simulink model "thermal_stress_control_gpu"  (R2025b)
settings: Solver=FixedStepDiscrete  StartTime=0.0  StopTime=40.0  FixedStep=0.05  RelTol=1e-3
undefined symbols (not defined in the file or in its folder): DiscIntNeverNeededParam
settings Model: Creator=fbetancourt  LastModifiedBy=fbetancourt

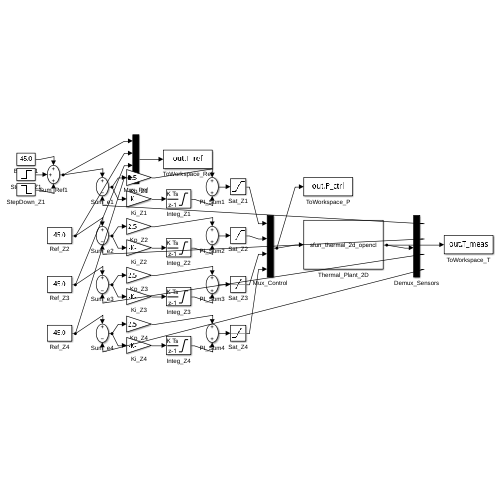
[thumbnail: Simulink's stored preview of the top-level diagram]
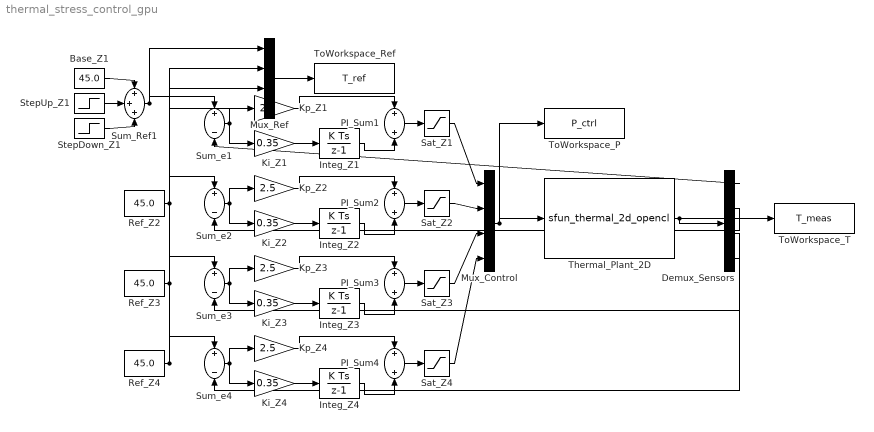
== system thermal_stress_control_gpu ==
  Base_Z1 : Constant  Value=45.0  SampleTime=0.05
  Demux_Sensors : Demux
  Integ_Z{1..4} (4 alike) : DiscreteIntegrator  SampleTime=0.05  LimitOutput=on  UpperSaturationLimit=100.0  LowerSaturationLimit=0.0  ICPrevOutput=DiscIntNeverNeededParam  ICPrevScaledInput=DiscIntNeverNeededParam
  Ki_Z{1..4} (4 alike) : Gain  Gain=0.35
  Kp_Z{1..4} (4 alike) : Gain  Gain=2.5
  Mux_Control : Mux
  Mux_Ref : Mux
  PI_Sum{1..4} (4 alike) : Sum
  Ref_Z2 : Constant  Value=45.0  SampleTime=0.05
  Ref_Z3 : Constant  Value=45.0  SampleTime=0.05
  Ref_Z4 : Constant  Value=45.0  SampleTime=0.05
  Sat_Z{1..4} (4 alike) : Saturate  UpperLimit=100.0  LowerLimit=0.0
  StepDown_Z1 : Step  Time=24.0  Before=0.0  After=-65.0  SampleTime=0.05
  StepUp_Z1 : Step  Time=8.0  Before=0.0  After=65.0  SampleTime=0.05
  Sum_Ref1 : Sum  Inputs=+++
  Sum_e{1..4} (4 alike) : Sum  Inputs=+-
  Thermal_Plant_2D : S-Function  FunctionName=sfun_thermal_2d_opencl  SFunctionDeploymentMode=off  EnableBusSupport=off
  ToWorkspace_P : ToWorkspace  VariableName=P_ctrl  SampleTime=0.05
  ToWorkspace_Ref : ToWorkspace  VariableName=T_ref  SampleTime=0.05
  ToWorkspace_T : ToWorkspace  VariableName=T_meas  SampleTime=0.05
  wires:
  Mux_Control/1 -> Thermal_Plant_2D/1, ToWorkspace_P/1
  Thermal_Plant_2D/1 -> Demux_Sensors/1, ToWorkspace_T/1
  Base_Z1/1 -> Sum_Ref1/1
  StepUp_Z1/1 -> Sum_Ref1/2
  StepDown_Z1/1 -> Sum_Ref1/3
  Sum_Ref1/1 -> Mux_Ref/1, Sum_e1/1
  Demux_Sensors/1 -> Sum_e1/2
  Sum_e1/1 -> Kp_Z1/1, Ki_Z1/1
  Ki_Z1/1 -> Integ_Z1/1
  Kp_Z1/1 -> PI_Sum1/1
  Integ_Z1/1 -> PI_Sum1/2
  PI_Sum1/1 -> Sat_Z1/1
  Sat_Z1/1 -> Mux_Control/1
  Ref_Z2/1 -> Mux_Ref/2, Sum_e2/1
  Demux_Sensors/2 -> Sum_e2/2
  Sum_e2/1 -> Kp_Z2/1, Ki_Z2/1
  Ki_Z2/1 -> Integ_Z2/1
  Kp_Z2/1 -> PI_Sum2/1
  Integ_Z2/1 -> PI_Sum2/2
  PI_Sum2/1 -> Sat_Z2/1
  Sat_Z2/1 -> Mux_Control/2
  Ref_Z3/1 -> Mux_Ref/3, Sum_e3/1
  Demux_Sensors/3 -> Sum_e3/2
  Sum_e3/1 -> Kp_Z3/1, Ki_Z3/1
  Ki_Z3/1 -> Integ_Z3/1
  Kp_Z3/1 -> PI_Sum3/1
  Integ_Z3/1 -> PI_Sum3/2
  PI_Sum3/1 -> Sat_Z3/1
  Sat_Z3/1 -> Mux_Control/3
  Ref_Z4/1 -> Mux_Ref/4, Sum_e4/1
  Demux_Sensors/4 -> Sum_e4/2
  Sum_e4/1 -> Kp_Z4/1, Ki_Z4/1
  Ki_Z4/1 -> Integ_Z4/1
  Kp_Z4/1 -> PI_Sum4/1
  Integ_Z4/1 -> PI_Sum4/2
  PI_Sum4/1 -> Sat_Z4/1
  Sat_Z4/1 -> Mux_Control/4
  Mux_Ref/1 -> ToWorkspace_Ref/1
